simulink model "DynamicMomentInertia_TestModel"  (R2014a)
settings: Solver=ode45  StartTime=0.0  StopTime=10.0  RelTol=1e-3
libraries: rocket_dynamic_data_library x2
settings Model: Creator=scorpii  LastModifiedBy=scorpii

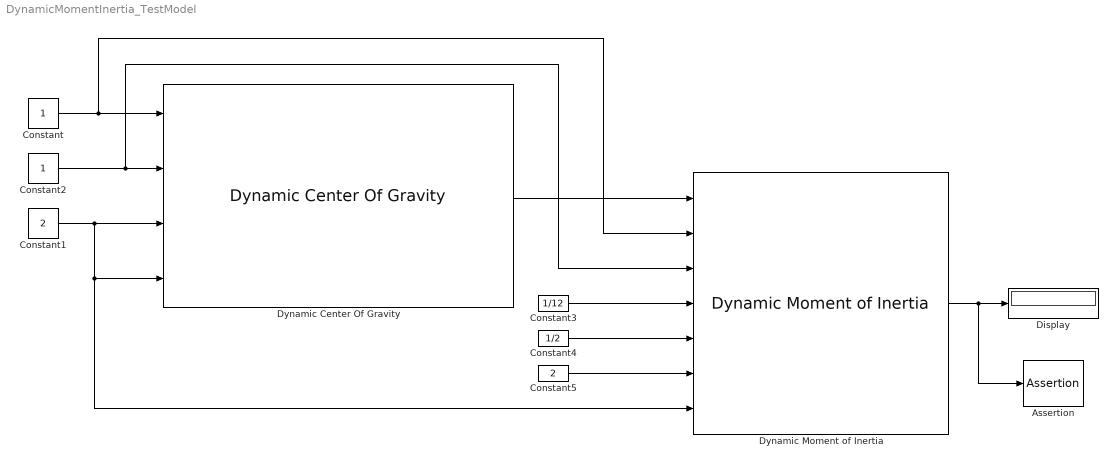
== system DynamicMomentInertia_TestModel ==
  Assertion : Assertion
  Constant : Constant
  Constant1 : Constant  Value=2
  Constant2 : Constant
  Constant3 : Constant  Value=1/12
  Constant4 : Constant  Value=1/2
  Constant5 : Constant  Value=2
  Display : Display
  Dynamic Center Of Gravity : rocket_dynamic_data_library/Dynamic Center Of Gravity
  Dynamic Moment of Inertia : rocket_dynamic_data_library/Dynamic Moment of Inertia
  wires:
  Constant/1 -> Dynamic Center Of Gravity/1, Dynamic Moment of Inertia/2
  Constant1/1 -> Dynamic Moment of Inertia/7, Dynamic Center Of Gravity/4, Dynamic Center Of Gravity/3
  Dynamic Center Of Gravity/1 -> Dynamic Moment of Inertia/1
  Constant2/1 -> Dynamic Moment of Inertia/3, Dynamic Center Of Gravity/2
  Constant3/1 -> Dynamic Moment of Inertia/4
  Constant4/1 -> Dynamic Moment of Inertia/5
  Constant5/1 -> Dynamic Moment of Inertia/6
  Dynamic Moment of Inertia/1 -> Assertion/1, Display/1
